simulink model "SMA_displacementIn_PC2_spring"  (R2018a)
settings: Solver=ode15s  StartTime=0.0  StopTime=20  RelTol=1e-9  AbsTol=1e-9  EnableMultiTasking=on
libraries: simulink x1
settings Model: Creator=Gianluca  LastModifiedBy=tim
settings SolverCC: AutoScaleAbsTol=off
settings DataIOCC: LimitDataPoints=on  SaveFormat=Array
settings OptimizationCC: LifeSpan=inf
settings DebuggingCC: UnderspecifiedInitializationDetection=Classic  MergeDetectMultiDrivingBlocksExec=none  SolverPrmCheckMsg=warning  StateNameClashWarn=warning  SFUnexpectedBacktrackingDiag=warning  SFNoUnconditionalDefaultTransitionDiag=warning  SFExecutionAtInitializationDiag=none
settings HardwareCC: ProdBitPerPointer=32  ProdBitPerSizeT=32  ProdBitPerPtrDiffT=32  ProdLargestAtomicFloat=None  ProdIntDivRoundTo=Undefined  ProdEndianess=Unspecified  ProdWordSize=32  ProdHWDeviceType=32-bit Generic
settings ModelReferenceCC: PropagateSignalLabelsOutOfModel=off
settings CodeAppCC: StateflowObjectComments=on
settings GRTTargetCC: TargetLangStandard=C89/C90 (ANSI)  GeneratePreprocessorConditionals=Disable all
settings ConfigComp: CovMetricSettings=dw  CovHtmlReporting=on  CovSaveCumulativeToWorkspaceVar=on  CovSaveSingleToWorkspaceVar=on  CovExternalEMLEnable=off

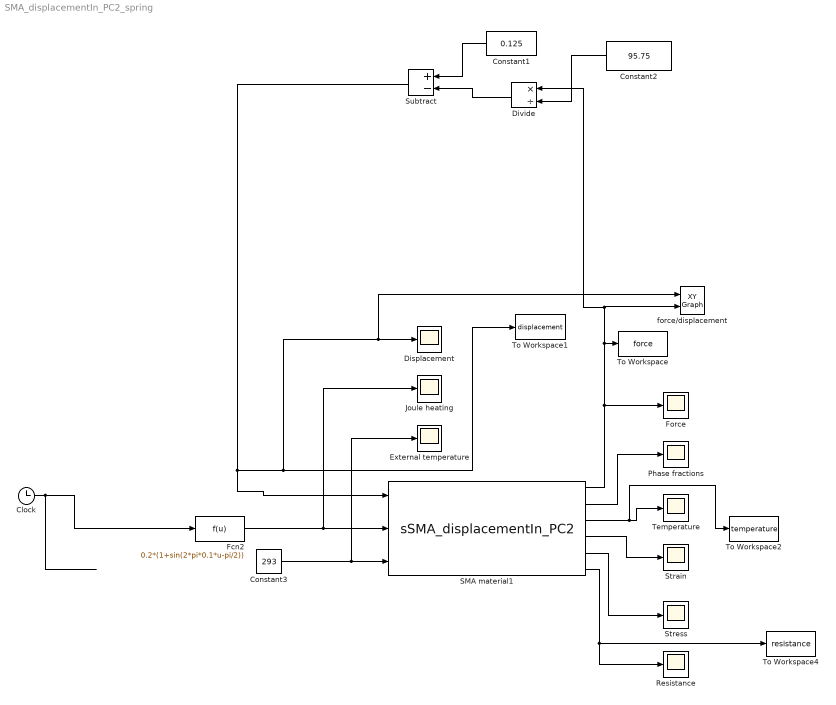
== system SMA_displacementIn_PC2_spring ==
  Clock : Clock
  Constant1 : Constant  Value=0.125
  Constant2 : Constant  Value=95.75
  Constant3 : Constant  Value=293
  Displacement : Scope
  Divide : Product  Inputs=*/
  External temperature : Scope
  Fcn2 : Fcn  Expr=0.2*(1+sin(2*pi*0.1*u-pi/2))
  Force : Scope
  Joule heating : Scope
  Phase fractions : Scope
  Resistance : Scope
  SMA material1 : M-S-Function  FunctionName=sSMA_displacementIn_PC2  Parameters=params_PC2, initConds_PC2
      mask Display:
      | color('black');
      | patch(3*[-1 1 1 -1],1.1*[-1 -1 1 1],[1 1 1]);
      | patch([-1.6 -0.8],[-0.9 0.3],[0 0 0]);
      | patch([-0.8 1.2],[0.3 0.3],[0 0 0]);
      | patch([1.6 0.8],[0.9 -0.3],[0 0 0]);
      | patch([0.8 -1.2],[-0.3 -0.3],[0 0 0]);
      | disp('SMA');
      | 
      | color('blue');
      | port_label('input', 1, 'y [m]','texmode','on');
      | port_label('input', 2, 'J [W]','texmode','on');
      | port_label('input', 3, 'T_E [K]','texmode','on');
      | 
      | color('red');
      | port_label('output', 1, 'F [N]','texmode','on');
      | port_label('output', 2, 'x_+, x_-, x_A [-]','texmode','on');
      | port_label('output', 3, 'T [K]','texmode','on');
      | port_label('output', 4, '\epsilon [-]','texmode','on');
      | port_label('output', 5, '\sigma [Pa]','texmode','on');
      | port_label('output', 6, 'R [\Omega]','texmode','on');
  Strain : Scope
  Stress : Scope
  Subtract : Sum  Inputs=+-
  Temperature : Scope
  To Workspace : ToWorkspace  VariableName=force  SampleTime=-1
  To Workspace1 : ToWorkspace  VariableName=displacement  SampleTime=-1
  To Workspace2 : ToWorkspace  VariableName=temperature  SampleTime=-1
  To Workspace4 : ToWorkspace  VariableName=resistance  SampleTime=-1
  force/displacement : simulink/Sinks/XY Graph  xmin=0.1  xmax=0.106  ymin=0  ymax=2.5  st=-1
  wires:
  Fcn2/1 -> Joule heating/1, SMA material1/2
  Constant3/1 -> SMA material1/3, External temperature/1
  SMA material1/2 -> Phase fractions/1
  SMA material1/3 -> To Workspace2/1, Temperature/1
  SMA material1/4 -> Strain/1
  SMA material1/5 -> Stress/1
  SMA material1/6 -> To Workspace4/1, Resistance/1
  SMA material1/1 -> To Workspace/1, Divide/1, force/displacement/2, Force/1
  Clock/1 -> Fcn2/1
  Constant1/1 -> Subtract/1
  Divide/1 -> Subtract/2
  Constant2/1 -> Divide/2
  Subtract/1 -> SMA material1/1, force/displacement/1, Displacement/1, To Workspace1/1
